simulink model "rudderAngle"  (Simulink 7.9)
settings: Solver=ode45  StartTime=0.0  StopTime=6.0  RelTol=1e-3
values from neighbouring files (symbols this model uses):
  A = 0.002    [params.m]
  v = 100    [params.m]
libraries: simulink x2
settings Model: Creator=dave  LastModifiedBy=dave

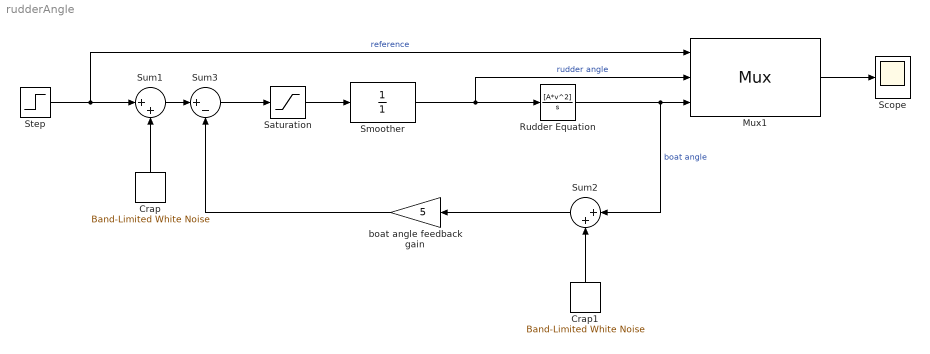
== system rudderAngle ==
  Crap : simulink/Sources/Band-Limited White Noise  Cov=[0.1]  Ts=0.1  seed=[23341]
  Crap1 : simulink/Sources/Band-Limited White Noise  Cov=[0.1]  Ts=0.1  seed=[23341]
  Mux1 : Mux  Inputs=3
      settings: DisplayOption=signals
  Rudder Equation : TransferFcn  Numerator=[A*v^2]  Denominator=[1 0]
  Saturation : Saturate  UpperLimit=25  LowerLimit=-25
  Scope : Scope
      settings: ShowLegends=on  TimeRange=6  YMin=-1.5  YMax=2
  Smoother : TransferFcn  Denominator=[0 1]
  Step : Step  After=40  SampleTime=0
  Sum1 : Sum  Inputs=|++
  Sum2 : Sum  Inputs=|++
  Sum3 : Sum  Inputs=|+-
  boat angle feedback gain : Gain  Gain=5
  wires:
  Saturation/1 -> Smoother/1
  Sum3/1 -> Saturation/1
  boat angle feedback gain/1 -> Sum3/2
  Smoother/1 -> Rudder Equation/1, Mux1/2  "rudder angle"
  Rudder Equation/1 -> Mux1/3, Sum2/1  "boat angle"
  Mux1/1 -> Scope/1
  Step/1 -> Sum1/1, Mux1/1  "reference"
  Crap/1 -> Sum1/2
  Sum1/1 -> Sum3/1
  Crap1/1 -> Sum2/2
  Sum2/1 -> boat angle feedback gain/1
